simulink model "Test_Pattern_Generator"  (R2013b)
settings: Solver=ode45  StartTime=0.0  StopTime=1500  RelTol=1e-3
InitFcn:
  | %% DSPBuilder Start
  | alt_dspbuilder_update_model(bdroot)
  | %% DSPBuilder End
libraries: allblocks_alteradspbuilder2 x106, simulink x4
(part 2 of 2)

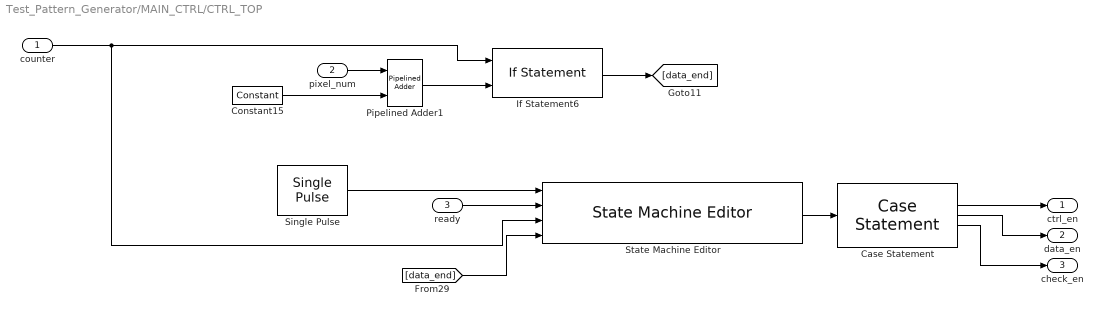
== system Test_Pattern_Generator/MAIN_CTRL/CTRL_TOP ==
  counter : Inport
  pixel_num : Inport  Port=2
  ready : Inport  Port=3
  Case Statement : allblocks_alteradspbuilder2/Case Statement  numOutputs=5  case_expression=0,1,2,4  formatted_case_expression=000,001,010,100  BusType=Unsigned Integer  bwl=3  bwr=0  pipeline=off  pipeline_display=0  hasDefault=on
  Constant15 : allblocks_alteradspbuilder2/Constant  mask_cst=4  BusType=Unsigned Integer  bwl=24  bwr=0  roundMode=Truncate  satMode=Wrap  SpecifyClock=off  allowFloatingPointOverride=on  logOutputs=off  logFile=E:\FPGA\SOC\Quartus\quartus\dsp_builder\design\VIP_LIB\Test_Pattern_Generator\tb_Test_Pattern_Generator\Test%5FPattern%5FGenerator_MAIN%5FCTRL_CTRL%5FTOP_Constant15.fixedpointlog
  If Statement6 : allblocks_alteradspbuilder2/If Statement  user_inputs=2  if_expression=a=b  BusType=Unsigned Integer  bwl=24  bwr=0  pipeline_display=1  use_else_output=off  use_elseif_input=off
  Pipelined Adder1 : allblocks_alteradspbuilder2/Pipelined Adder  BusType=Unsigned Integer  bwl=24  bwr=0  pipeline=2  pipeline_display=2  AddSubDirection=ADD  use_cin=off  use_ovl=off  use_addsub=off  use_ena=off  use_aclr=off  or_aclr_inputs=on
  Single Pulse : allblocks_alteradspbuilder2/Single Pulse  signal_type=Step Down  impulse_width=1  delay=1  SpecifyClock=off  use_ena=off  use_sclr=off
  State Machine Editor : allblocks_alteradspbuilder2/State Machine Editor  entityName=StateMachineEditor_import  use_dynamic_feedthrough_data=on  inNames=reset ready counter data_end  inBwls=1 1 24 1  inBwrs="0  0  0  0"  inTypes=b b s b  inDelayed="0  1  0  1"  outNames=state  outBwls=3  outBwrs=0  outTypes=s  n_input_port=4  n_output_port=1  array_clocks=clock  xmlmapfile=E:\FPGA\SOC\Quartus\quartus\dsp_builder\lib\SimgenCMap.xml  vofile=DSPBuilder_Test_Pattern_Generator_import\StateMachineEditor.vo  use_systemC_model=off  is_megacore=off  smf_variation=|
      | /*                                                                         
      | WARNING: Do NOT edit the input and output ports in this file in a text     
      | editor if you plan to continue editing the block that represents it in     
      | the Block Editor! File corruption is VERY likely to occur.                 
      | Copyright (C) 1991-2013 Altera Corporation                                 
      | Your use of Altera Corporation's design tools, logic functions             
      | and other software and tools, and its AMPP partner logic                   
      | functions, and any output files from any of the foregoing                  
      | (including device programming or simulation files), and any                
      | associated documentation or information are expressly subject              
      | to the terms and conditions of the Altera Program License                  
      | Subscription Agreement, Altera MegaCore Function License                   
      | Agreement, or other applicable license agreement, including,               
      | without limitation, that your use is for the sole purpose of               
      | programming logic devices manufactured by Altera and sold by               
      | Altera or its authorized distributors.  Please refer to the                
      | applicable agreement for further details.                                  
      | Generated by Quartus II Version 13.1.0 Build 162 10/23/2013 SJ Full Version
      | Created on Wed Feb 11 09:38:56 2015                                        
      | */                                                                         
      | VERSION = "3.0";                                                           
      | HEADER                                                                     
      | (                                                                          
      | 	GENERAL{                                                                  
      | 		RMODE = "S";                                                             
      | 		RA_LEVEL = "H";                                                          
      | 		HOPT = "VHDL";                                                           
      | 	}                                                                         
      | 	SPORT{                                                                    
      | 		NAME = "clock";                                                          
      | 		PTYPE = "CI";                                                            
      | 		REG = "N";                                                               
      | 		OUTS = "N";                                                              
      | 	}                                                                         
      | 	SPORT{                                                                    
      | 		NAME = "reset";                                                          
      | 		PTYPE = "RI";                                                            
      | 		REG = "N";                                                               
      | 		OUTS = "N";                                                              
      | 	}                                                                         
      | 	SPORT{                                                                    
      | 		NAME = "ready";                                                          
      | 		PTYPE = "OI";                                                            
      | 		REG = "N";                                                               
      | 		OUTS = "N";                                                              
      | 	}                                                                         
      | 	SPORT{                                                                    
      | 		NAME = "counter[23:0]";                                                  
      | 		PTYPE = "OI";                                                            
      | 		REG = "N";                                                               
      | 		OUTS = "N";                                                              
      | 	}                                                                         
      | 	SPORT{                                                                    
      | 		NAME = "data_end";                                                       
      | 		PTYPE = "OI";                                                            
      | 		REG = "N";                                                               
      | 		OUTS = "N";                                                              
      | 	}                                                                         
      | 	SPORT{                                                                    
      | 		NAME = "state[2:0]";                                                     
      | 		PTYPE = "OU";                                                            
      | 		REG = "N";                                                               
      | 		OUTS = "C";                                                              
      | 	}                                                                         
      | 	STATE{                                                                    
      | 		NAME = "CTRL";                                                           
      | 		STYPE = "NR";                                                            
      | 		PT = (256,328);                                                          
      | 		OUTP = "state[2:0]";                                                     
      | 		OUT_VALUE = "1";                                                         
      | 		COND = "";                                                               
      | 	}                                                                         
      | 	STATE{                                                                    
      | 		NAME = "DATA";                                                           
      | 		STYPE = "NR";                                                            
      | 		PT = (568,336);                                                          
      | 		OUTP = "state[2:0]";                                                     
      | 		OUT_VALUE = "2";                                                         
      | 		COND = "";                                                               
      | 	}                                                                         
      | 	STATE{                                                                    
      | 		NAME = "IDLE";                                                           
      | 		STYPE = "RE";                                                            
      | 		PT = (416,136);                                                          
      | 		OUTP = "state[2:0]";                                                     
      | 		OUT_VALUE = "0";                                                         
      | 		COND = "counter!=0";                                                     
      | 		OUTP = "state[2:0]";                                                     
      | 		OUT_VALUE = "4";                                                         
      | 		COND = "counter==0";                                                     
      | 	}                                                                         
      | 	TRANS{                                                                    
      | 		SSTATE = "CTRL";                                                         
      | 		DSTATE = "IDLE";                                                         
      | 		EQ = "(ready==0)|(counter==3)";                                          
      | 		PT = (301,338);                                                          
      | 		PT = (348,287);                                                          
      | 		PT = (395,236);                                                          
      | 		PT = (444,184);                                                          
      | 		PT = (343,292);                                                          
      | 	}                                                                         
      | 	TRANS{                                                                    
      | 		SSTATE = "IDLE";                                                         
      | 		DSTATE = "DATA";                                                         
      | 		EQ = "(ready==1)&(counter>3)";                                           
      | 		PT = (465,160);                                                          
      | 		PT = (502,220);                                                          
      | 		PT = (539,280);                                                          
      | 		PT = (577,341);                                                          
      | 		PT = (496,214);                                                          
      | 	}                                                                         
      | 	TRANS{                                                                    
      | 		SSTATE = "DATA";                                                         
      | 		DSTATE = "IDLE";                                                         
      | 		EQ = "(ready==0)|((ready==1)&(data_end==1))";                            
      | 		PT = (567,360);                                                          
      | 		PT = (530,300);                                                          
      | 		PT = (493,240);                                                          
      | 		PT = (455,179);                                                          
      | 		PT = (535,306);                                                          
      | 	}                                                                         
      | 	TRANS{                                                                    
      | 		SSTATE = "IDLE";                                                         
      | 		DSTATE = "CTRL";                                                         
      | 		EQ = "(ready==1)&(counter<=3)";                                          
      | 		PT = (424,179);                                                          
      | 		PT = (383,232);                                                          
      | 		PT = (342,285);                                                          
      | 		PT = (301,338);                                                          
      | 		PT = (387,228);                                                          
      | 	}                                                                         
      | 	TRANS{                                                                    
      | 		SSTATE = "IDLE";                                                         
      | 		DSTATE = "IDLE";                                                         
      | 		EQ = "ready==0";                                                         
      | 		PT = (458,143);                                                          
      | 		PT = (494,143);                                                          
      | 		PT = (494,178);                                                          
      | 		PT = (458,178);                                                          
      | 		PT = (499,158);                                                          
      | 	}                                                                         
      | 	TRANS{                                                                    
      | 		SSTATE = "DATA";                                                         
      | 		DSTATE = "DATA";                                                         
      | 		EQ = "(ready==1)&(data_end==0)";                                         
      | 		PT = (610,343);                                                          
      | 		PT = (646,343);                                                          
      | 		PT = (646,378);                                                          
      | 		PT = (610,378);                                                          
      | 		PT = (651,358);                                                          
      | 	}                                                                         
      | 	TRANS{                                                                    
      | 		SSTATE = "CTRL";                                                         
      | 		DSTATE = "CTRL";                                                         
      | 		EQ = "(ready==1)&(counter<3)";                                           
      | 		PT = (298,335);                                                          
      | 		PT = (334,335);                                                          
      | 		PT = (334,370);                                                          
      | 		PT = (298,370);                                                          
      | 		PT = (339,350);                                                          
      | 	}                                                                         
      | )                                                                          
      | END
  ctrl_en : Outport
  data_en : Outport  Port=2
  check_en : Outport  Port=3
  wires:
  ready/1 -> State Machine Editor/2
  counter/1 -> State Machine Editor/3, If Statement6/1
  Single Pulse/1 -> State Machine Editor/1
  State Machine Editor/1 -> Case Statement/1
  Case Statement/2 -> ctrl_en/1
  Case Statement/3 -> data_en/1
  [data_end] -> State Machine Editor/4
  If Statement6/1 -> [data_end]
  pixel_num/1 -> Pipelined Adder1/1
  Constant15/1 -> Pipelined Adder1/2
  Pipelined Adder1/1 -> If Statement6/2
  Case Statement/4 -> check_en/1

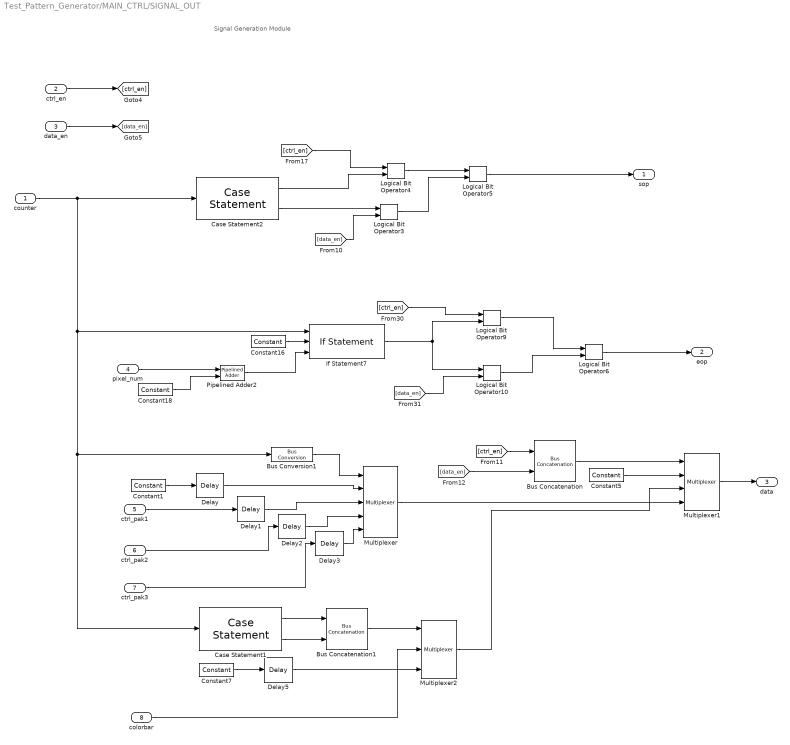
== system Test_Pattern_Generator/MAIN_CTRL/SIGNAL_OUT ==
  note: Signal Generation Module
  counter : Inport
  ctrl_en : Inport  Port=2
  data_en : Inport  Port=3
  pixel_num : Inport  Port=4
  ctrl_pak1 : Inport  Port=5
  ctrl_pak2 : Inport  Port=6
  ctrl_pak3 : Inport  Port=7
  colorbar : Inport  Port=8
  Bus Concatenation : allblocks_alteradspbuilder2/Bus Concatenation  isSigned=off  awidth=1  bwidth=1  pipeline_display=0
  Bus Concatenation1 : allblocks_alteradspbuilder2/Bus Concatenation  isSigned=off  awidth=1  bwidth=1  pipeline_display=0
  Bus Conversion1 : allblocks_alteradspbuilder2/Bus Conversion  BusType=Unsigned Integer  ibwl=24  ibwr=1  bwl=2  bwr=1  bitToConnectToOutputLSB=0  round=off  saturate=off  pipeline_display=0
  Case Statement1 : allblocks_alteradspbuilder2/Case Statement  numOutputs=2  case_expression=4  formatted_case_expression=0000000000000100  BusType=Unsigned Integer  bwl=16  bwr=0  pipeline=off  pipeline_display=0  hasDefault=on
  Case Statement2 : allblocks_alteradspbuilder2/Case Statement  numOutputs=2  case_expression=0,4  formatted_case_expression=0000000000000000,0000000000000100  BusType=Unsigned Integer  bwl=16  bwr=0  pipeline=off  pipeline_display=0  hasDefault=off
  Constant1 : allblocks_alteradspbuilder2/Constant  mask_cst=15  BusType=Unsigned Integer  bwl=24  bwr=0  roundMode=Truncate  satMode=Wrap  SpecifyClock=off  allowFloatingPointOverride=on  logOutputs=off  logFile=E:\FPGA\SOC\Quartus\quartus\dsp_builder\design\VIP_LIB\Test_Pattern_Generator\tb_Test_Pattern_Generator\Test%5FPattern%5FGenerator_MAIN%5FCTRL_SIGNAL%5FOUT_Constant1.fixedpointlog
  Constant16 : allblocks_alteradspbuilder2/Constant  mask_cst=3  BusType=Unsigned Integer  bwl=16  bwr=0  roundMode=Truncate  satMode=Wrap  SpecifyClock=off  allowFloatingPointOverride=on  logOutputs=off  logFile=E:\FPGA\SOC\Quartus\quartus\dsp_builder\design\VIP_LIB\Test_Pattern_Generator\tb_Test_Pattern_Generator\Test%5FPattern%5FGenerator_MAIN%5FCTRL_SIGNAL%5FOUT_Constant16.fixedpointlog
  Constant18 : allblocks_alteradspbuilder2/Constant  mask_cst=4  BusType=Unsigned Integer  bwl=24  bwr=0  roundMode=Truncate  satMode=Wrap  SpecifyClock=off  allowFloatingPointOverride=on  logOutputs=off  logFile=E:\FPGA\SOC\Quartus\quartus\dsp_builder\design\VIP_LIB\Test_Pattern_Generator\tb_Test_Pattern_Generator\Test%5FPattern%5FGenerator_MAIN%5FCTRL_SIGNAL%5FOUT_Constant18.fixedpointlog
  Constant5 : allblocks_alteradspbuilder2/Constant  mask_cst=0  BusType=Unsigned Integer  bwl=24  bwr=0  roundMode=Truncate  satMode=Wrap  SpecifyClock=off  allowFloatingPointOverride=on  logOutputs=off  logFile=E:\FPGA\SOC\Quartus\quartus\dsp_builder\design\VIP_LIB\Test_Pattern_Generator\tb_Test_Pattern_Generator\Test%5FPattern%5FGenerator_MAIN%5FCTRL_SIGNAL%5FOUT_Constant5.fixedpointlog
  Constant7 : allblocks_alteradspbuilder2/Constant  mask_cst=0  BusType=Unsigned Integer  bwl=24  bwr=0  roundMode=Truncate  satMode=Wrap  SpecifyClock=off  allowFloatingPointOverride=on  logOutputs=off  logFile=E:\FPGA\SOC\Quartus\quartus\dsp_builder\design\VIP_LIB\Test_Pattern_Generator\tb_Test_Pattern_Generator\Test%5FPattern%5FGenerator_MAIN%5FCTRL_SIGNAL%5FOUT_Constant7.fixedpointlog
  Delay : allblocks_alteradspbuilder2/Delay  pipeline=1  pipeline_display=1  ClockPhase=1  use_ena=off  use_sclr=off  allowFloatingPointOverride=on  logOutputs=off  logFile=E:\FPGA\SOC\Quartus\quartus\dsp_builder\design\VIP_LIB\Test_Pattern_Generator\tb_Test_Pattern_Generator\Test%5FPattern%5FGenerator_MAIN%5FCTRL_SIGNAL%5FOUT_Delay.fixedpointlog  use_init=off  reset_value=15
  Delay1 : allblocks_alteradspbuilder2/Delay  pipeline=1  pipeline_display=1  ClockPhase=1  use_ena=off  use_sclr=off  allowFloatingPointOverride=on  logOutputs=off  logFile=E:\FPGA\SOC\Quartus\quartus\dsp_builder\design\VIP_LIB\Test_Pattern_Generator\tb_Test_Pattern_Generator\Test%5FPattern%5FGenerator_MAIN%5FCTRL_SIGNAL%5FOUT_Delay1.fixedpointlog  use_init=off  reset_value=2
  Delay2 : allblocks_alteradspbuilder2/Delay  pipeline=1  pipeline_display=1  ClockPhase=1  use_ena=off  use_sclr=off  allowFloatingPointOverride=on  logOutputs=off  logFile=E:\FPGA\SOC\Quartus\quartus\dsp_builder\design\VIP_LIB\Test_Pattern_Generator\tb_Test_Pattern_Generator\Test%5FPattern%5FGenerator_MAIN%5FCTRL_SIGNAL%5FOUT_Delay2.fixedpointlog  use_init=off  reset_value=0
  Delay3 : allblocks_alteradspbuilder2/Delay  pipeline=1  pipeline_display=1  ClockPhase=1  use_ena=off  use_sclr=off  allowFloatingPointOverride=on  logOutputs=off  logFile=E:\FPGA\SOC\Quartus\quartus\dsp_builder\design\VIP_LIB\Test_Pattern_Generator\tb_Test_Pattern_Generator\Test%5FPattern%5FGenerator_MAIN%5FCTRL_SIGNAL%5FOUT_Delay3.fixedpointlog  use_init=off  reset_value=2
  Delay5 : allblocks_alteradspbuilder2/Delay  pipeline=1  pipeline_display=1  ClockPhase=1  use_ena=off  use_sclr=off  allowFloatingPointOverride=on  logOutputs=off  logFile=E:\FPGA\SOC\Quartus\quartus\dsp_builder\design\VIP_LIB\Test_Pattern_Generator\tb_Test_Pattern_Generator\Test%5FPattern%5FGenerator_MAIN%5FCTRL_SIGNAL%5FOUT_Delay5.fixedpointlog  use_init=off  reset_value=2
  If Statement7 : allblocks_alteradspbuilder2/If Statement  user_inputs=3  if_expression=(a=b)|(a=c)  BusType=Unsigned Integer  bwl=24  bwr=0  pipeline_display=1  use_else_output=off  use_elseif_input=off
  Logical Bit Operator{3..4,9..10} (4 alike) : allblocks_alteradspbuilder2/Logical Bit Operator  LogicalOperator=AND  user_inputs=2  pipeline_display=0
  Logical Bit Operator5 : allblocks_alteradspbuilder2/Logical Bit Operator  LogicalOperator=OR  user_inputs=2  pipeline_display=0
  Logical Bit Operator6 : allblocks_alteradspbuilder2/Logical Bit Operator  LogicalOperator=OR  user_inputs=2  pipeline_display=0
  Multiplexer : allblocks_alteradspbuilder2/Multiplexer  numInputs=4  pipeline=0  oneHot=off  pipeline_display=0  use_ena=on  use_aclr=off  allowFloatingPointOverride=off  logOutputs=off  logFile=E:\FPGA\SOC\Quartus\quartus\dsp_builder\design\VIP_LIB\Test_Pattern_Generator\tb_Test_Pattern_Generator\Test%5FPattern%5FGenerator_MAIN%5FCTRL_SIGNAL%5FOUT_Multiplexer.fixedpointlog
  Multiplexer1 : allblocks_alteradspbuilder2/Multiplexer  numInputs=3  pipeline=0  oneHot=off  pipeline_display=0  use_ena=off  use_aclr=off  allowFloatingPointOverride=off  logOutputs=off  logFile=E:\FPGA\SOC\Quartus\quartus\dsp_builder\design\VIP_LIB\Test_Pattern_Generator\tb_Test_Pattern_Generator\Test%5FPattern%5FGenerator_MAIN%5FCTRL_SIGNAL%5FOUT_Multiplexer1.fixedpointlog
  Multiplexer2 : allblocks_alteradspbuilder2/Multiplexer  numInputs=2  pipeline=0  oneHot=on  pipeline_display=0  use_ena=off  use_aclr=off  allowFloatingPointOverride=off  logOutputs=off  logFile=E:\FPGA\SOC\Quartus\quartus\dsp_builder\design\VIP_LIB\Test_Pattern_Generator\tb_Test_Pattern_Generator\Test%5FPattern%5FGenerator_MAIN%5FCTRL_SIGNAL%5FOUT_Multiplexer2.fixedpointlog
  Pipelined Adder2 : allblocks_alteradspbuilder2/Pipelined Adder  BusType=Unsigned Integer  bwl=24  bwr=0  pipeline=2  pipeline_display=2  AddSubDirection=ADD  use_cin=off  use_ovl=off  use_addsub=off  use_ena=off  use_aclr=off  or_aclr_inputs=on
  sop : Outport
  eop : Outport  Port=2
  data : Outport  Port=3
  wires:
  Logical Bit Operator5/1 -> sop/1
  [ctrl_en] -> Logical Bit Operator4/1
  Case Statement2/1 -> Logical Bit Operator4/2
  Logical Bit Operator4/1 -> Logical Bit Operator5/1
  counter/1 -> If Statement7/1, Case Statement1/1, Bus Conversion1/1, Case Statement2/1
  Logical Bit Operator6/1 -> eop/1
  Case Statement2/2 -> Logical Bit Operator3/1
  [data_en] -> Logical Bit Operator3/2
  Logical Bit Operator3/1 -> Logical Bit Operator5/2
  [ctrl_en] -> Logical Bit Operator9/1
  Logical Bit Operator9/1 -> Logical Bit Operator6/1
  [data_en] -> Logical Bit Operator10/2
  Logical Bit Operator10/1 -> Logical Bit Operator6/2
  Constant16/1 -> If Statement7/2
  Constant18/1 -> Pipelined Adder2/2
  Pipelined Adder2/1 -> If Statement7/3
  If Statement7/1 -> Logical Bit Operator10/1, Logical Bit Operator9/2
  Bus Conversion1/1 -> Multiplexer/1
  Multiplexer/1 -> Multiplexer1/4
  Constant1/1 -> Delay/1
  Bus Concatenation/1 -> Multiplexer1/1
  [ctrl_en] -> Bus Concatenation/1
  [data_en] -> Bus Concatenation/2
  Constant5/1 -> Multiplexer1/2
  Multiplexer2/1 -> Multiplexer1/3
  Delay/1 -> Multiplexer/2
  Delay1/1 -> Multiplexer/3
  Delay2/1 -> Multiplexer/4
  Delay3/1 -> Multiplexer/5
  Case Statement1/1 -> Bus Concatenation1/1
  Case Statement1/2 -> Bus Concatenation1/2
  Bus Concatenation1/1 -> Multiplexer2/1
  Constant7/1 -> Delay5/1
  Delay5/1 -> Multiplexer2/3
  colorbar/1 -> Multiplexer2/2
  ctrl_en/1 -> [ctrl_en]
  data_en/1 -> [data_en]
  Multiplexer1/1 -> data/1
  ctrl_pak1/1 -> Delay1/1
  ctrl_pak2/1 -> Delay2/1
  ctrl_pak3/1 -> Delay3/1
  pixel_num/1 -> Pipelined Adder2/1
